simulink model "PV_model_subsystem_R2017a"  (R2017a)
settings: Solver=ode45  StartTime=0.0  StopTime=1  MaxStep=1e-6  RelTol=1e-3
values from neighbouring files (symbols this model uses):
  a = 1.01185853243    [cs6u320p_data.mat]    (also in kc85t_data.mat = 1.07116014082)
  Gn = 1000    [cs6u320p_data.mat]    (also in kc85t_data.mat)
  Ipvn = 9.27160885018    [cs6u320p_data.mat]    (also in kc85t_data.mat = 5.34348225514)
  Iscn = 9.26    [cs6u320p_data.mat]    (also in kc85t_data.mat = 5.34)
  k = 1.3806503e-23    [cs6u320p_data.mat]    (also in kc85t_data.mat)
  Ki = 0.0049078    [cs6u320p_data.mat]    (also in kc85t_data.mat = 0.00212)
  Kv = -0.14043    [cs6u320p_data.mat]    (also in kc85t_data.mat = -0.0821)
  Ns = 72    [cs6u320p_data.mat]    (also in kc85t_data.mat = 36)
  q = 1.60217646e-19    [cs6u320p_data.mat]    (also in kc85t_data.mat)
  Rp = 258.214084743    [cs6u320p_data.mat]    (also in kc85t_data.mat = 439.463329238)
  Rs = 0.32    [cs6u320p_data.mat]    (also in kc85t_data.mat = 0.277)
  Tn = 298.15    [cs6u320p_data.mat]    (also in kc85t_data.mat)
  Vocn = 45.3    [cs6u320p_data.mat]    (also in kc85t_data.mat = 21.7)
libraries: powerlib x9, simulink x1
settings Model: Creator=Marcos  LastModifiedBy=Marcos

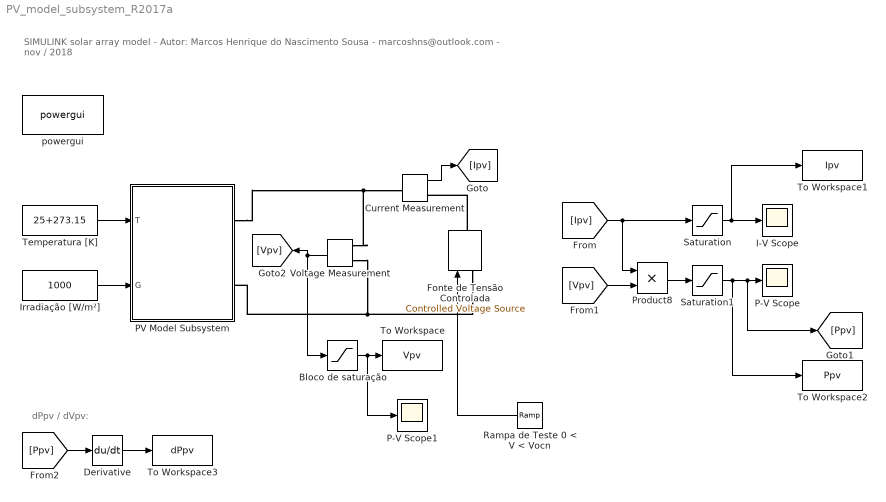
== system PV_model_subsystem_R2017a ==
  note: dPpv / dVpv:
  note: SIMULINK solar array model - Autor: Marcos Henrique do Nascimento Sousa - marcoshns@outlook.com - nov / 2018
  Bloco de saturação : Saturate  UpperLimit=350  LowerLimit=0
  Current Measurement : powerlib/Measurements/Current Measurement  PhasorSimulation=off  OutputType=Complex  PSBequivalent=0
  Derivative : Derivative
  Fonte de Tensão Controlada : powerlib/Electrical Sources/Controlled Voltage Source  Initialize=on  Source_Type=DC  Amplitude=0  Phase=0  Frequency=0  Measurements=None
  I-V Scope : Scope
  Irradiação [W/m²] : Constant  Value=1000
  P-V Scope : Scope
  P-V Scope1 : Scope
  PV Model Subsystem : Subsystem
  Product8 : Product
  "Rampa de Teste 0 < V < Vocn " : simulink/Sources/Ramp  slope=Vocn  start=0  X0=0
  Saturation : Saturate  UpperLimit=100  LowerLimit=0
  Saturation1 : Saturate  UpperLimit=350  LowerLimit=0
  Temperatura [K] : Constant  Value=25+273.15
  To Workspace : ToWorkspace  VariableName=Vpv  SampleTime=-1
  To Workspace1 : ToWorkspace  VariableName=Ipv  SampleTime=-1
  To Workspace2 : ToWorkspace  VariableName=Ppv  SampleTime=-1
  To Workspace3 : ToWorkspace  VariableName=dPpv  SampleTime=-1
  Voltage Measurement : powerlib/Measurements/Voltage Measurement  PhasorSimulation=off  OutputType=Complex  PSBequivalent=0
  powergui : powerlib/powergui  Priority=1  SimulationMode=Discrete  SampleTime=1e-3  frequency=60  Iterations=50  frequencyindice=0  Pbase=100e6  ErrMax=1e-4  UnitsV=kV  UnitsW=MW  buscounter=0  FunctionMessages=off  echomessages=off  EnableUseOfTLC=off  CurrentSourceSwitches=off  DisableSnubberDevices=off  DisableRonSwitches=off  DisableVfSwitches=off  DisplayEquations=off  SolverType=Tustin/Backward Euler (TBE)  Interpol=off  ExternalGateDelay=off  methode=off  Ts=100  x0status=blocks  SPID=on  SwTol=0  HookPort=off  RestoreLinks=warning  ResistiveCurrentMeasurement=off  Frange=[0:2:500]  Ylog=off  Xlog=on  ShowGrid=off  save=off  variable=ZData  structure=0  ZoomFFT=off  StartTime=0.0  cycles=1  DisplayStyle=1  fundamental=60  FreqAxis=off  MaxFrequency=1000  frequencyindicesteady=1  RmsSteady=1  display=off
  wires:
  Saturation/1 -> To Workspace1/1, I-V Scope/1
  Product8/1 -> Saturation1/1
  Saturation1/1 -> To Workspace2/1, [Ppv], P-V Scope/1
  Temperatura [K]/1 -> PV Model Subsystem/1(T)
  Irradiação [W/m²]/1 -> PV Model Subsystem/2(G)
  Current Measurement/1 -> [Ipv]
  Voltage Measurement/1 -> Bloco de saturação/1, [Vpv]
  [Ipv] -> Product8/1, Saturation/1
  [Vpv] -> Product8/2
  [Ppv] -> Derivative/1
  Derivative/1 -> To Workspace3/1
  Bloco de saturação/1 -> P-V Scope1/1, To Workspace/1
  "Rampa de Teste 0 < V < Vocn "/1 -> Fonte de Tensão Controlada/1
  connections:
  Voltage Measurement/LConn1 -- PV Model Subsystem/RConn1 -- Current Measurement/LConn1
  Fonte de Tensão Controlada/LConn1 -- Voltage Measurement/LConn2 -- PV Model Subsystem/RConn2
  Fonte de Tensão Controlada/RConn1 -- Current Measurement/RConn1

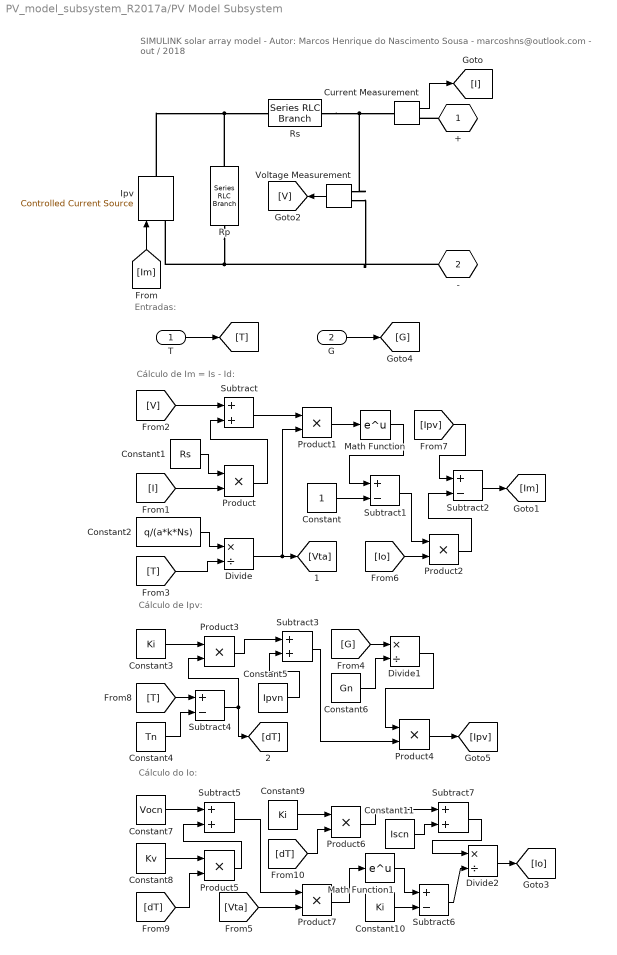
== system PV_model_subsystem_R2017a/PV Model Subsystem ==
  note: Cálculo de Im = Is - Id:
  note: Cálculo de Ipv:
  note: Entradas:
  note: Cálculo do Io:
  note: SIMULINK solar array model - Autor: Marcos Henrique do Nascimento Sousa - marcoshns@outlook.com - out / 2018
  T : Inport
  G : Inport  Port=2
  Constant : Constant
  Constant1 : Constant  Value=Rs
  Constant10 : Constant  Value=Ki
  Constant11 : Constant  Value=Iscn
  Constant2 : Constant  Value=q/(a*k*Ns)
  Constant3 : Constant  Value=Ki
  Constant4 : Constant  Value=Tn
  Constant5 : Constant  Value=Ipvn
  Constant6 : Constant  Value=Gn
  Constant7 : Constant  Value=Vocn
  Constant8 : Constant  Value=Kv
  Constant9 : Constant  Value=Ki
  Current Measurement : powerlib/Measurements/Current Measurement  PhasorSimulation=off  OutputType=Complex  PSBequivalent=0
  Divide : Product  Inputs=*/
  Divide1 : Product  Inputs=*/
  Divide2 : Product  Inputs=*/
  Ipv : powerlib/Electrical Sources/Controlled Current Source  Initialize=on  Source_Type=DC  Amplitude=0  Phase=0  Frequency=0  Measurements=None
  Math Function : Math  SaturateOnIntegerOverflow=on
  Math Function1 : Math  SaturateOnIntegerOverflow=on
  Product{,1..7} (8 alike) : Product
  Rp : powerlib/Elements/Series RLC Branch  LConnTagsString=__new0  RConnTagsString=__new0  BranchType=R  Resistance=Rp  Inductance=1e-3  SetiL0=off  InitialCurrent=0  Capacitance=1e-6  Setx0=off  InitialVoltage=0  Measurements=None
  Rs : powerlib/Elements/Series RLC Branch  LConnTagsString=__new0  RConnTagsString=__new0  BranchType=R  Resistance=Rs  Inductance=1e-3  SetiL0=off  InitialCurrent=0  Capacitance=1e-6  Setx0=off  InitialVoltage=0  Measurements=None
  Subtract{,3,5,7} (4 alike) : Sum
  Subtract{1..2,4,6} (4 alike) : Sum  Inputs=+-
  Voltage Measurement : powerlib/Measurements/Voltage Measurement  PhasorSimulation=off  OutputType=Complex  PSBequivalent=0
  + : PMIOPort  Tag=PMCPort  Port=1  Side=Right
  - : PMIOPort  Tag=PMCPort  Port=2  Side=Right
  wires:
  Constant11/1 -> Subtract7/2
  Product6/1 -> Subtract7/1
  Subtract5/1 -> Product7/1
  Math Function1/1 -> Subtract6/1
  [Ipv] -> Subtract2/1
  [dT] -> Product6/2
  [I] -> Product/2
  [Im] -> Ipv/1
  [dT] -> Product5/2
  Product/1 -> Subtract/2
  Product1/1 -> Math Function/1
  G/1 -> [G]
  [Vta] -> Product7/2
  [V] -> Subtract/1
  [T] -> Divide/2
  Product3/1 -> Subtract3/1
  Constant4/1 -> Subtract4/2
  Constant7/1 -> Subtract5/1
  Subtract3/1 -> Product4/2
  Constant9/1 -> Product6/1
  Math Function/1 -> Subtract1/1
  Constant1/1 -> Product/1
  [Io] -> Product2/2
  Product5/1 -> Subtract5/2
  Subtract4/1 -> [dT], Product3/2
  [T] -> Subtract4/1
  Constant5/1 -> Subtract3/2
  Product2/1 -> Subtract2/2
  Subtract6/1 -> Divide2/2
  Subtract2/1 -> [Im]
  Divide2/1 -> [Io]
  Constant6/1 -> Divide1/2
  T/1 -> [T]
  Product4/1 -> [Ipv]
  Product7/1 -> Math Function1/1
  Constant10/1 -> Subtract6/2
  Divide1/1 -> Product4/1
  Constant8/1 -> Product5/1
  Subtract1/1 -> Product2/1
  Constant3/1 -> Product3/1
  Constant2/1 -> Divide/1
  Subtract/1 -> Product1/1
  Subtract7/1 -> Divide2/1
  [G] -> Divide1/1
  Constant/1 -> Subtract1/2
  Divide/1 -> [Vta], Product1/2
  Current Measurement/1 -> [I]
  Voltage Measurement/1 -> [V]
  connections:
  Rp/RConn1 -- Ipv/LConn1 -- Voltage Measurement/LConn2 -- -/RConn1
  Ipv/RConn1 -- Rs/LConn1 -- Rp/LConn1
  Voltage Measurement/LConn1 -- Current Measurement/LConn1 -- Rs/RConn1
  +/RConn1 -- Current Measurement/RConn1
